simulink model "generic_uservehicle_truck"  (Simulink 8.7)
settings: Solver=ode45  StartTime=0.0  StopTime=inf  RelTol=1e-3
(part 2 of 3)

== system generic_uservehicle_truck/TruckMaker/Vehicle/User Vehicle (ModelMgr)/PowerTrain ==
  note: When replacing the entire powertrain,
      | be sure to disable the IPG powertrain model by using the powertrain
      | model 'Model Manager off' in the vehicle GUI.
  note: <Your model here>
  Sync_In : Inport
  Vhcl.Wheel.PT : Inport  Port=2
  VhclCtrl.PT : Inport  Port=3
  BusCreator : BusCreator  Inputs=70
  Demux : Demux  Outputs=70
  PowerTrain : S-Function  FunctionName=TM_Sfun  Parameters='PowerTrain'  SFunctionDeploymentMode=off  EnableBusSupport=off
  PowerTrainUpd : S-Function  FunctionName=TM_Sfun  Parameters='PowerTrainUpd'  SFunctionDeploymentMode=off  EnableBusSupport=off
  Sync_Out : Outport
  wires:
  Demux/70 -> BusCreator/70  "PT IF WFR2 Trq_BrakeReg_max"
  Demux/69 -> BusCreator/69  "PT IF WFR2 Trq_BrakeReg"
  Demux/68 -> BusCreator/68  "PT IF WFR2 Trq_Supp2WC"
  Demux/67 -> BusCreator/67  "PT IF WFR2 Trq_Drive"
  Demux/66 -> BusCreator/66  "PT IF WFR2 Trq_B2W"
  Demux/65 -> BusCreator/65  "PT IF WFR2 rotv"
  Demux/64 -> BusCreator/64  "PT IF WFR2 rot"
  Demux/63 -> BusCreator/63  "PT IF WFL2 Trq_BrakeReg_max"
  Demux/62 -> BusCreator/62  "PT IF WFL2 Trq_BrakeReg"
  Demux/61 -> BusCreator/61  "PT IF WFL2 Trq_Supp2WC"
  Demux/60 -> BusCreator/60  "PT IF WFL2 Trq_Drive"
  Demux/59 -> BusCreator/59  "PT IF WFL2 Trq_B2W"
  Demux/58 -> BusCreator/58  "PT IF WFL2 rotv"
  Demux/57 -> BusCreator/57  "PT IF WFL2 rot"
  Demux/56 -> BusCreator/56  "PT IF WRR2 Trq_BrakeReg_max"
  Demux/55 -> BusCreator/55  "PT IF WRR2 Trq_BrakeReg"
  Demux/54 -> BusCreator/54  "PT IF WRR2 Trq_Supp2WC"
  Demux/53 -> BusCreator/53  "PT IF WRR2 Trq_Drive"
  Demux/52 -> BusCreator/52  "PT IF WRR2 Trq_B2W"
  Demux/51 -> BusCreator/51  "PT IF WRR2 rotv"
  Demux/50 -> BusCreator/50  "PT IF WRR2 rot"
  Demux/49 -> BusCreator/49  "PT IF WRL2 Trq_BrakeReg_max"
  Demux/48 -> BusCreator/48  "PT IF WRL2 Trq_BrakeReg"
  Demux/47 -> BusCreator/47  "PT IF WRL2 Trq_Supp2WC"
  Demux/46 -> BusCreator/46  "PT IF WRL2 Trq_Drive"
  Demux/45 -> BusCreator/45  "PT IF WRL2 Trq_B2W"
  Demux/44 -> BusCreator/44  "PT IF WRL2 rotv"
  Demux/43 -> BusCreator/43  "PT IF WRL2 rot"
  Demux/42 -> BusCreator/42  "PT IF WRR Trq_BrakeReg_max"
  Demux/41 -> BusCreator/41  "PT IF WRR Trq_BrakeReg"
  Demux/40 -> BusCreator/40  "PT IF WRR Trq_Supp2WC"
  Demux/39 -> BusCreator/39  "PT IF WRR Trq_Drive"
  Demux/38 -> BusCreator/38  "PT IF WRR Trq_B2W"
  Demux/37 -> BusCreator/37  "PT IF WRR rotv"
  Demux/36 -> BusCreator/36  "PT IF WRR rot"
  Demux/35 -> BusCreator/35  "PT IF WRL Trq_BrakeReg_max"
  Demux/34 -> BusCreator/34  "PT IF WRL Trq_BrakeReg"
  Demux/33 -> BusCreator/33  "PT IF WRL Trq_Supp2WC"
  Demux/32 -> BusCreator/32  "PT IF WRL Trq_Drive"
  Demux/31 -> BusCreator/31  "PT IF WRL Trq_B2W"
  Demux/30 -> BusCreator/30  "PT IF WRL rotv"
  Demux/29 -> BusCreator/29  "PT IF WRL rot"
  Demux/28 -> BusCreator/28  "PT IF WFR Trq_BrakeReg_max"
  Demux/27 -> BusCreator/27  "PT IF WFR Trq_BrakeReg"
  Demux/26 -> BusCreator/26  "PT IF WFR Trq_Supp2WC"
  Demux/25 -> BusCreator/25  "PT IF WFR Trq_Drive"
  Demux/24 -> BusCreator/24  "PT IF WFR Trq_B2W"
  Demux/23 -> BusCreator/23  "PT IF WFR rotv"
  Demux/22 -> BusCreator/22  "PT IF WFR rot"
  Demux/21 -> BusCreator/21  "PT IF WFL Trq_BrakeReg_max"
  Demux/20 -> BusCreator/20  "PT IF WFL Trq_BrakeReg"
  Demux/19 -> BusCreator/19  "PT IF WFL Trq_Supp2WC"
  Demux/18 -> BusCreator/18  "PT IF WFL Trq_Drive"
  Demux/17 -> BusCreator/17  "PT IF WFL Trq_B2W"
  Demux/16 -> BusCreator/16  "PT IF WFL rotv"
  Demux/15 -> BusCreator/15  "PT IF WFL rot"
  Demux/14 -> BusCreator/14  "PT IF DL_iDiff_mean"
  Demux/13 -> BusCreator/13  "PT IF Trq_Supp2BdyEng y"
  Demux/12 -> BusCreator/12  "PT IF Trq_Supp2BdyEng x"
  Demux/11 -> BusCreator/11  "PT IF Trq_Supp2Bdy1B z"
  Demux/10 -> BusCreator/10  "PT IF Trq_Supp2Bdy1B y"
  Demux/9 -> BusCreator/9  "PT IF Trq_Supp2Bdy1B x"
  Demux/8 -> BusCreator/8  "PT IF Trq_Supp2Bdy1 z"
  Demux/7 -> BusCreator/7  "PT IF Trq_Supp2Bdy1 y"
  Demux/6 -> BusCreator/6  "PT IF Trq_Supp2Bdy1 x"
  Demux/5 -> BusCreator/5  "PT IF Engine_rotv"
  Demux/4 -> BusCreator/4  "PT IF GearNo"
  Demux/3 -> BusCreator/3  "PT IF OperationError"
  Demux/2 -> BusCreator/2  "PT IF OperationState"
  Demux/1 -> BusCreator/1  "PT IF Ignition"
  BusCreator/1 -> PowerTrainUpd/2
  PowerTrain/2 -> Demux/1
  Sync_In/1 -> PowerTrain/1
  PowerTrainUpd/1 -> Sync_Out/1
  PowerTrain/1 -> PowerTrainUpd/1  "Sync"
  VhclCtrl.PT/1 -> PowerTrain/3
  Vhcl.Wheel.PT/1 -> PowerTrain/2

== system generic_uservehicle_truck/TruckMaker/Vehicle/User Vehicle (ModelMgr)/VehicleSource_ModelMgr ==
  u : Inport
  Compare : RelationalOperator  Operator=~=  OutDataTypeStr=boolean  ZeroCross=off  InputSameDT=on
  Constant : Constant  DisableCoverage=on  Value=const  OutDataTypeStr=Inherit: Inherit via back propagation
  y : Outport
  wires:
  u/1 -> Compare/1
  Constant/1 -> Compare/2
  Compare/1 -> y/1

== system generic_uservehicle_truck/TruckMaker/Vehicle/IPG Vehicle/Brake/CreateBus Vhcl.Wheel.PT ==
  In : Inport
  BusCreator : BusCreator  Inputs=40
  Demux : Demux  Outputs=40
  Out : Outport
  wires:
  Demux/40 -> BusCreator/40  "Vhcl Trq_DriveSrc_trg d7"
  Demux/39 -> BusCreator/39  "Vhcl Trq_DriveSrc_trg d6"
  Demux/38 -> BusCreator/38  "Vhcl Trq_DriveSrc_trg d5"
  Demux/37 -> BusCreator/37  "Vhcl Trq_DriveSrc_trg d4"
  Demux/36 -> BusCreator/36  "Vhcl Trq_DriveSrc_trg d3"
  Demux/35 -> BusCreator/35  "Vhcl Trq_DriveSrc_trg d2"
  Demux/34 -> BusCreator/34  "Vhcl Trq_DriveSrc_trg d1"
  Demux/33 -> BusCreator/33  "Vhcl Trq_DriveSrc_trg d0"
  Demux/32 -> BusCreator/32  "Vhcl Wheel FR2 WhlBearing"
  Demux/31 -> BusCreator/31  "Vhcl Wheel FR2 Trq_T2W"
  Demux/30 -> BusCreator/30  "Vhcl Wheel FR2 Trq_BrakeReg_trg"
  Demux/29 -> BusCreator/29  "Vhcl Wheel FR2 Trq_Brake"
  Demux/28 -> BusCreator/28  "Vhcl Wheel FL2 WhlBearing"
  Demux/27 -> BusCreator/27  "Vhcl Wheel FL2 Trq_T2W"
  Demux/26 -> BusCreator/26  "Vhcl Wheel FL2 Trq_BrakeReg_trg"
  Demux/25 -> BusCreator/25  "Vhcl Wheel FL2 Trq_Brake"
  Demux/24 -> BusCreator/24  "Vhcl Wheel RR2 WhlBearing"
  Demux/23 -> BusCreator/23  "Vhcl Wheel RR2 Trq_T2W"
  Demux/22 -> BusCreator/22  "Vhcl Wheel RR2 Trq_BrakeReg_trg"
  Demux/21 -> BusCreator/21  "Vhcl Wheel RR2 Trq_Brake"
  Demux/20 -> BusCreator/20  "Vhcl Wheel RL2 WhlBearing"
  Demux/19 -> BusCreator/19  "Vhcl Wheel RL2 Trq_T2W"
  Demux/18 -> BusCreator/18  "Vhcl Wheel RL2 Trq_BrakeReg_trg"
  Demux/17 -> BusCreator/17  "Vhcl Wheel RL2 Trq_Brake"
  Demux/16 -> BusCreator/16  "Vhcl Wheel RR WhlBearing"
  Demux/15 -> BusCreator/15  "Vhcl Wheel RR Trq_T2W"
  Demux/14 -> BusCreator/14  "Vhcl Wheel RR Trq_BrakeReg_trg"
  Demux/13 -> BusCreator/13  "Vhcl Wheel RR Trq_Brake"
  Demux/12 -> BusCreator/12  "Vhcl Wheel RL WhlBearing"
  Demux/11 -> BusCreator/11  "Vhcl Wheel RL Trq_T2W"
  Demux/10 -> BusCreator/10  "Vhcl Wheel RL Trq_BrakeReg_trg"
  Demux/9 -> BusCreator/9  "Vhcl Wheel RL Trq_Brake"
  Demux/8 -> BusCreator/8  "Vhcl Wheel FR WhlBearing"
  Demux/7 -> BusCreator/7  "Vhcl Wheel FR Trq_T2W"
  Demux/6 -> BusCreator/6  "Vhcl Wheel FR Trq_BrakeReg_trg"
  Demux/5 -> BusCreator/5  "Vhcl Wheel FR Trq_Brake"
  Demux/4 -> BusCreator/4  "Vhcl Wheel FL WhlBearing"
  Demux/3 -> BusCreator/3  "Vhcl Wheel FL Trq_T2W"
  Demux/2 -> BusCreator/2  "Vhcl Wheel FL Trq_BrakeReg_trg"
  Demux/1 -> BusCreator/1  "Vhcl Wheel FL Trq_Brake"
  BusCreator/1 -> Out/1
  In/1 -> Demux/1

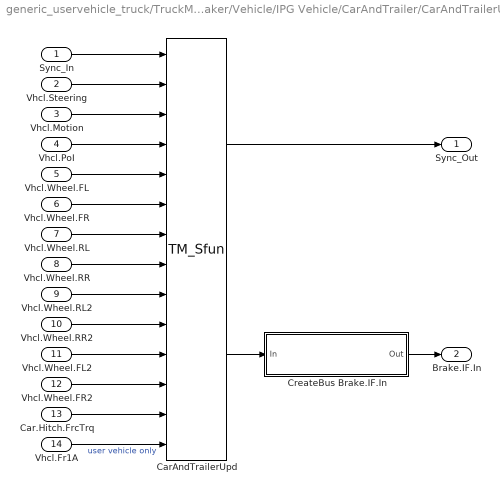
== system generic_uservehicle_truck/TruckMaker/Vehicle/IPG Vehicle/CarAndTrailer/CarAndTrailerUpd ==
  Sync_In : Inport
  Vhcl.Steering : Inport  Port=2
  Vhcl.Motion : Inport  Port=3
  Vhcl.PoI : Inport  Port=4
  Vhcl.Wheel.FL : Inport  Port=5
  Vhcl.Wheel.FR : Inport  Port=6
  Vhcl.Wheel.RL : Inport  Port=7
  Vhcl.Wheel.RR : Inport  Port=8
  Vhcl.Wheel.RL2 : Inport  Port=9
  Vhcl.Wheel.RR2 : Inport  Port=10
  Vhcl.Wheel.FL2 : Inport  Port=11
  Vhcl.Wheel.FR2 : Inport  Port=12
  Car.Hitch.FrcTrq : Inport  Port=13
  Vhcl.Fr1A : Inport  Port=14
  CarAndTrailerUpd : S-Function  FunctionName=TM_Sfun  Parameters='CarAndTrUpd'  SFunctionDeploymentMode=off  EnableBusSupport=off
  CreateBus Brake.IF.In : Subsystem
  Sync_Out : Outport
  Brake.IF.In : Outport  Port=2
  wires:
  Vhcl.Fr1A/1 -> CarAndTrailerUpd/14  "user vehicle only"
  Vhcl.Wheel.RL2/1 -> CarAndTrailerUpd/9
  Vhcl.Wheel.RR2/1 -> CarAndTrailerUpd/10
  Vhcl.Wheel.FL2/1 -> CarAndTrailerUpd/11
  Vhcl.Wheel.FR2/1 -> CarAndTrailerUpd/12
  Car.Hitch.FrcTrq/1 -> CarAndTrailerUpd/13
  Vhcl.Wheel.RR/1 -> CarAndTrailerUpd/8
  Vhcl.Wheel.RL/1 -> CarAndTrailerUpd/7
  Vhcl.Wheel.FR/1 -> CarAndTrailerUpd/6
  Vhcl.Wheel.FL/1 -> CarAndTrailerUpd/5
  Vhcl.Steering/1 -> CarAndTrailerUpd/2
  Vhcl.Motion/1 -> CarAndTrailerUpd/3
  Vhcl.PoI/1 -> CarAndTrailerUpd/4
  CarAndTrailerUpd/2 -> CreateBus Brake.IF.In/1(In)
  CreateBus Brake.IF.In/1(Out) -> Brake.IF.In/1
  CarAndTrailerUpd/1 -> Sync_Out/1
  Sync_In/1 -> CarAndTrailerUpd/1

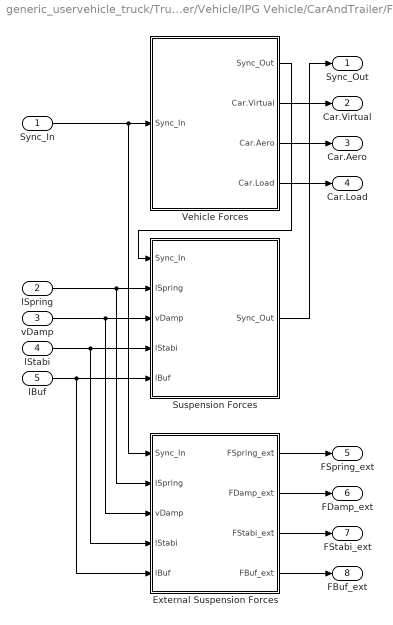
== system generic_uservehicle_truck/TruckMaker/Vehicle/IPG Vehicle/CarAndTrailer/Forces ==
  Sync_In : Inport
  lSpring : Inport  Port=2
  vDamp : Inport  Port=3
  lStabi : Inport  Port=4
  lBuf : Inport  Port=5
  External Suspension Forces : Subsystem
  Suspension Forces : Subsystem
  Vehicle Forces : Subsystem
  Sync_Out : Outport
  Car.Virtual : Outport  Port=2
  Car.Aero : Outport  Port=3
  Car.Load : Outport  Port=4
  FSpring_ext : Outport  Port=5
  FDamp_ext : Outport  Port=6
  FStabi_ext : Outport  Port=7
  FBuf_ext : Outport  Port=8
  wires:
  Sync_In/1 -> External Suspension Forces/1(Sync_In), Vehicle Forces/1(Sync_In)
  Vehicle Forces/2(Car.Virtual) -> Car.Virtual/1
  Vehicle Forces/3(Car.Aero) -> Car.Aero/1
  Vehicle Forces/4(Car.Load) -> Car.Load/1
  lSpring/1 -> Suspension Forces/2(lSpring), External Suspension Forces/2(lSpring)
  External Suspension Forces/2(FDamp_ext) -> FDamp_ext/1
  vDamp/1 -> Suspension Forces/3(vDamp), External Suspension Forces/3(vDamp)
  lStabi/1 -> Suspension Forces/4(lStabi), External Suspension Forces/4(lStabi)
  External Suspension Forces/3(FStabi_ext) -> FStabi_ext/1
  External Suspension Forces/1(FSpring_ext) -> FSpring_ext/1
  lBuf/1 -> Suspension Forces/5(lBuf), External Suspension Forces/5(lBuf)
  External Suspension Forces/4(FBuf_ext) -> FBuf_ext/1
  Vehicle Forces/1(Sync_Out) -> Suspension Forces/1(Sync_In)
  Suspension Forces/1(Sync_Out) -> Sync_Out/1

== system generic_uservehicle_truck/TruckMaker/Vehicle/IPG Vehicle/CarAndTrailer/Kinematics ==
  Sync_In : Inport
  Steer.IF : Inport  Port=2
  Kinematics : S-Function  FunctionName=TM_Sfun  Parameters='Kinematics'  SFunctionDeploymentMode=off  EnableBusSupport=off
  TireFL.In : Terminator
  TireFR.In : Terminator
  TireRL.In : Terminator
  TireRR.In : Terminator
  Sync_Out : Outport
  lSpring : Outport  Port=2
  vDamp : Outport  Port=3
  lStabi : Outport  Port=4
  lBuf : Outport  Port=5
  wires:
  Kinematics/8 -> lStabi/1
  Kinematics/2 -> TireFL.In/1
  Kinematics/3 -> TireFR.In/1
  Kinematics/4 -> TireRL.In/1
  Kinematics/5 -> TireRR.In/1
  Kinematics/6 -> lSpring/1
  Kinematics/7 -> vDamp/1
  Sync_In/1 -> Kinematics/1
  Kinematics/1 -> Sync_Out/1
  Steer.IF/1 -> Kinematics/2
  Kinematics/9 -> lBuf/1

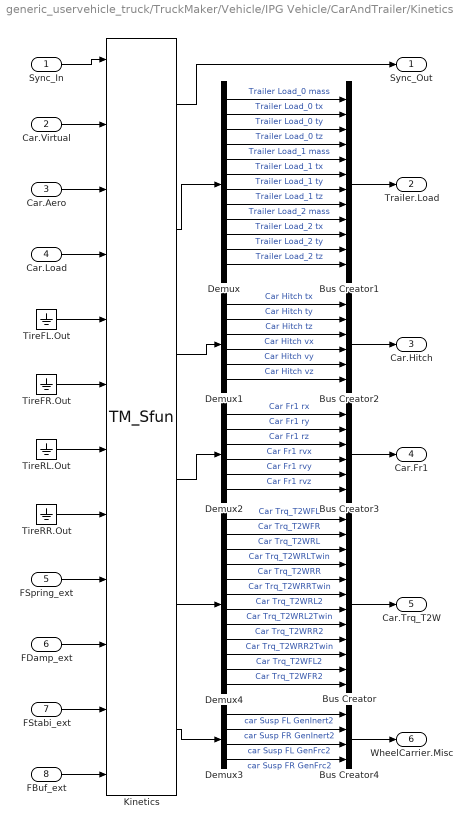
== system generic_uservehicle_truck/TruckMaker/Vehicle/IPG Vehicle/CarAndTrailer/Kinetics ==
  Sync_In : Inport
  Car.Virtual : Inport  Port=2
  Car.Aero : Inport  Port=3
  Car.Load : Inport  Port=4
  FSpring_ext : Inport  Port=5
  FDamp_ext : Inport  Port=6
  FStabi_ext : Inport  Port=7
  FBuf_ext : Inport  Port=8
  Bus Creator : BusCreator  Inputs=12
  Bus Creator1 : BusCreator  Inputs=12
  Bus Creator2 : BusCreator  Inputs=6
  Bus Creator3 : BusCreator  Inputs=6
  Bus Creator4 : BusCreator  Inputs=4
  Demux : Demux  Outputs=12
  Demux1 : Demux  Outputs=6
  Demux2 : Demux  Outputs=6
  Demux3 : Demux
  Demux4 : Demux  Outputs=12
  Kinetics : S-Function  FunctionName=TM_Sfun  Parameters='Kinetics'  SFunctionDeploymentMode=off  EnableBusSupport=off
  TireFL.Out : Ground
  TireFR.Out : Ground
  TireRL.Out : Ground
  TireRR.Out : Ground
  Sync_Out : Outport
  Trailer.Load : Outport  Port=2
  Car.Hitch : Outport  Port=3
  Car.Fr1 : Outport  Port=4
  Car.Trq_T2W : Outport  Port=5
  WheelCarrier.Misc : Outport  Port=6
  wires:
  Demux4/12 -> Bus Creator/12  "Car Trq_T2WFR2"
  Demux4/11 -> Bus Creator/11  "Car Trq_T2WFL2"
  Sync_In/1 -> Kinetics/1
  Kinetics/1 -> Sync_Out/1
  Car.Aero/1 -> Kinetics/3
  Car.Virtual/1 -> Kinetics/2
  Bus Creator1/1 -> Trailer.Load/1
  Demux/1 -> Bus Creator1/1  "Trailer Load_0 mass"
  Demux/2 -> Bus Creator1/2  "Trailer Load_0 tx"
  Demux/3 -> Bus Creator1/3  "Trailer Load_0 ty"
  Demux/4 -> Bus Creator1/4  "Trailer Load_0 tz"
  Kinetics/2 -> Demux/1
  Demux/5 -> Bus Creator1/5  "Trailer Load_1 mass"
  Demux/6 -> Bus Creator1/6  "Trailer Load_1 tx"
  Demux/7 -> Bus Creator1/7  "Trailer Load_1 ty"
  Demux/8 -> Bus Creator1/8  "Trailer Load_1 tz"
  Demux/9 -> Bus Creator1/9  "Trailer Load_2 mass"
  Demux/10 -> Bus Creator1/10  "Trailer Load_2 tx"
  Demux/11 -> Bus Creator1/11  "Trailer Load_2 ty"
  Demux/12 -> Bus Creator1/12  "Trailer Load_2 tz"
  Demux1/1 -> Bus Creator2/1  "Car Hitch tx"
  Demux1/2 -> Bus Creator2/2  "Car Hitch ty"
  Demux1/3 -> Bus Creator2/3  "Car Hitch tz"
  Demux1/4 -> Bus Creator2/4  "Car Hitch vx"
  Demux1/5 -> Bus Creator2/5  "Car Hitch vy"
  Demux1/6 -> Bus Creator2/6  "Car Hitch vz"
  Kinetics/3 -> Demux1/1
  Bus Creator2/1 -> Car.Hitch/1
  Demux2/1 -> Bus Creator3/1  "Car Fr1 rx"
  Demux2/2 -> Bus Creator3/2  "Car Fr1 ry"
  Demux2/3 -> Bus Creator3/3  "Car Fr1 rz"
  Demux2/4 -> Bus Creator3/4  "Car Fr1 rvx"
  Demux2/5 -> Bus Creator3/5  "Car Fr1 rvy"
  Demux2/6 -> Bus Creator3/6  "Car Fr1 rvz"
  Bus Creator3/1 -> Car.Fr1/1
  Kinetics/4 -> Demux2/1
  Car.Load/1 -> Kinetics/4
  Demux3/1 -> Bus Creator4/1  "car Susp FL GenInert2"
  Demux3/2 -> Bus Creator4/2  "car Susp FR GenInert2"
  Demux3/3 -> Bus Creator4/3  "car Susp FL GenFrc2"
  Demux3/4 -> Bus Creator4/4  "car Susp FR GenFrc2"
  Bus Creator4/1 -> WheelCarrier.Misc/1
  Demux4/3 -> Bus Creator/3  "Car Trq_T2WRL"
  Demux4/2 -> Bus Creator/2  "Car Trq_T2WFR"
  Demux4/1 -> Bus Creator/1  "Car Trq_T2WFL"
  TireFL.Out/1 -> Kinetics/5
  TireFR.Out/1 -> Kinetics/6
  TireRL.Out/1 -> Kinetics/7
  TireRR.Out/1 -> Kinetics/8
  FSpring_ext/1 -> Kinetics/9
  FDamp_ext/1 -> Kinetics/10
  FStabi_ext/1 -> Kinetics/11
  Kinetics/6 -> Demux3/1
  Kinetics/5 -> Demux4/1
  Bus Creator/1 -> Car.Trq_T2W/1
  Demux4/9 -> Bus Creator/9  "Car Trq_T2WRR2"
  Demux4/10 -> Bus Creator/10  "Car Trq_T2WRR2Twin"
  Demux4/7 -> Bus Creator/7  "Car Trq_T2WRL2"
  Demux4/8 -> Bus Creator/8  "Car Trq_T2WRL2Twin"
  Demux4/5 -> Bus Creator/5  "Car Trq_T2WRR"
  Demux4/4 -> Bus Creator/4  "Car Trq_T2WRLTwin"
  Demux4/6 -> Bus Creator/6  "Car Trq_T2WRRTwin"
  FBuf_ext/1 -> Kinetics/12

== system generic_uservehicle_truck/TruckMaker/Vehicle/IPG Vehicle/CarAndTrailer/Steering ==
  note: When replacing the entire steering system,
      | be sure to disable the IPG steering model by using the steering
      | model 'Model Manager off' in the vehicle GUI.
  Sync_In : Inport
  VhclCtrl.Steering : Inport  Port=2
  Bus Creator1 : BusCreator  Inputs=16
  Bus Creator2 : BusCreator  Inputs=5
  Demux : Demux  Outputs=21
  Steering : S-Function  FunctionName=TM_Sfun  Parameters='Steering'  SFunctionDeploymentMode=off  EnableBusSupport=off
  Terminator : Terminator
  Sync_Out : Outport
  Steer.IF : Outport  Port=2
  wires:
  Demux/21 -> Bus Creator2/5  "Steering IF R Inert"
  Demux/20 -> Bus Creator2/4  "Steering IF R Frc"
  Demux/19 -> Bus Creator2/3  "Steering IF L Inert"
  Demux/18 -> Bus Creator2/2  "Steering IF L Frc"
  Demux/17 -> Bus Creator2/1  "Steering IF SteerByTrq"
  Demux/16 -> Bus Creator1/16  "Steering IF R iSteer2q"
  Demux/15 -> Bus Creator1/15  "Steering IF R qpp"
  Demux/14 -> Bus Creator1/14  "Steering IF R qp"
  Demux/13 -> Bus Creator1/13  "Steering IF R q"
  Demux/12 -> Bus Creator1/12  "Steering IF L iSteer2q"
  Demux/11 -> Bus Creator1/11  "Steering IF L qpp"
  Demux/10 -> Bus Creator1/10  "Steering IF L qp"
  Demux/9 -> Bus Creator1/9  "Steering IF L q"
  Demux/8 -> Bus Creator1/8  "Steering IF AssistTrqPin"
  Demux/7 -> Bus Creator1/7  "Steering IF AssistTrqCol"
  Demux/6 -> Bus Creator1/6  "Steering IF AssistFrc"
  Demux/5 -> Bus Creator1/5  "Steering IF TrqStatic"
  Demux/4 -> Bus Creator1/4  "Steering IF Trq"
  Demux/3 -> Bus Creator1/3  "Steering IF AngAcc"
  Demux/2 -> Bus Creator1/2  "Steering IF AngVel"
  Demux/1 -> Bus Creator1/1  "Steering IF Ang"
  Bus Creator1/1 -> Steer.IF/1
  Bus Creator2/1 -> Terminator/1  "Steer IF (in)"
  Sync_In/1 -> Steering/1
  Steering/1 -> Sync_Out/1
  VhclCtrl.Steering/1 -> Steering/2
  Steering/2 -> Demux/1

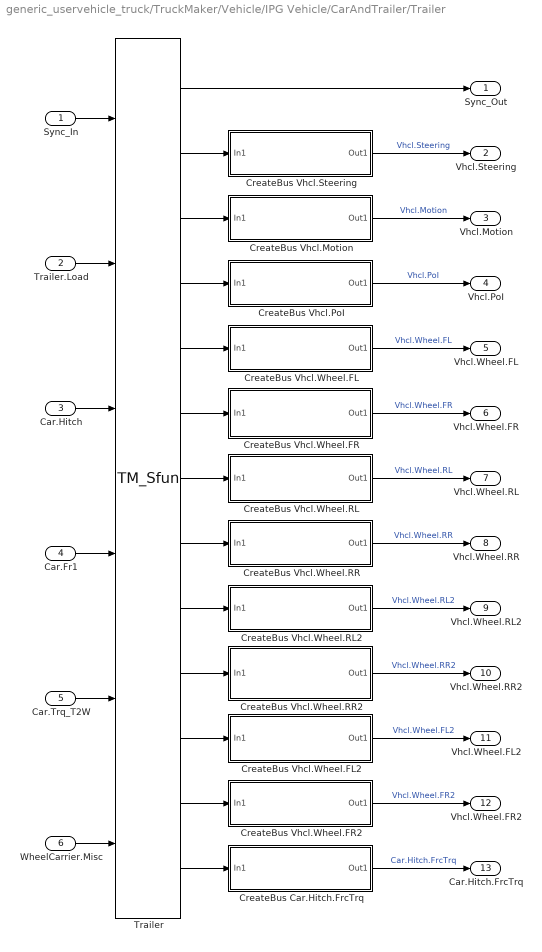
== system generic_uservehicle_truck/TruckMaker/Vehicle/IPG Vehicle/CarAndTrailer/Trailer ==
  Sync_In : Inport
  Trailer.Load : Inport  Port=2
  Car.Hitch : Inport  Port=3
  Car.Fr1 : Inport  Port=4
  Car.Trq_T2W : Inport  Port=5
  WheelCarrier.Misc : Inport  Port=6
  CreateBus Car.Hitch.FrcTrq : Subsystem
  CreateBus Vhcl.Motion : Subsystem
  CreateBus Vhcl.PoI : Subsystem
  CreateBus Vhcl.Steering : Subsystem
  CreateBus Vhcl.Wheel.FL : Subsystem
  CreateBus Vhcl.Wheel.FL2 : Subsystem
  CreateBus Vhcl.Wheel.FR : Subsystem
  CreateBus Vhcl.Wheel.FR2 : Subsystem
  CreateBus Vhcl.Wheel.RL : Subsystem
  CreateBus Vhcl.Wheel.RL2 : Subsystem
  CreateBus Vhcl.Wheel.RR : Subsystem
  CreateBus Vhcl.Wheel.RR2 : Subsystem
  Trailer : S-Function  FunctionName=TM_Sfun  Parameters='Trailer'  SFunctionDeploymentMode=off  EnableBusSupport=off
  Sync_Out : Outport
  Vhcl.Steering : Outport  Port=2
  Vhcl.Motion : Outport  Port=3
  Vhcl.PoI : Outport  Port=4
  Vhcl.Wheel.FL : Outport  Port=5
  Vhcl.Wheel.FR : Outport  Port=6
  Vhcl.Wheel.RL : Outport  Port=7
  Vhcl.Wheel.RR : Outport  Port=8
  Vhcl.Wheel.RL2 : Outport  Port=9
  Vhcl.Wheel.RR2 : Outport  Port=10
  Vhcl.Wheel.FL2 : Outport  Port=11
  Vhcl.Wheel.FR2 : Outport  Port=12
  Car.Hitch.FrcTrq : Outport  Port=13
  wires:
  CreateBus Vhcl.Wheel.RL2/1(Out1) -> Vhcl.Wheel.RL2/1  "Vhcl.Wheel.RL2"
  CreateBus Vhcl.Wheel.RR2/1(Out1) -> Vhcl.Wheel.RR2/1  "Vhcl.Wheel.RR2"
  CreateBus Vhcl.Wheel.FL2/1(Out1) -> Vhcl.Wheel.FL2/1  "Vhcl.Wheel.FL2"
  CreateBus Vhcl.Wheel.FR2/1(Out1) -> Vhcl.Wheel.FR2/1  "Vhcl.Wheel.FR2"
  Trailer/12 -> CreateBus Vhcl.Wheel.FR2/1(In1)
  Trailer/11 -> CreateBus Vhcl.Wheel.FL2/1(In1)
  Trailer/10 -> CreateBus Vhcl.Wheel.RR2/1(In1)
  Trailer/9 -> CreateBus Vhcl.Wheel.RL2/1(In1)
  CreateBus Vhcl.Wheel.FL/1(Out1) -> Vhcl.Wheel.FL/1  "Vhcl.Wheel.FL"
  CreateBus Vhcl.Wheel.FR/1(Out1) -> Vhcl.Wheel.FR/1  "Vhcl.Wheel.FR"
  CreateBus Vhcl.Wheel.RL/1(Out1) -> Vhcl.Wheel.RL/1  "Vhcl.Wheel.RL"
  CreateBus Vhcl.Wheel.RR/1(Out1) -> Vhcl.Wheel.RR/1  "Vhcl.Wheel.RR"
  Trailer/8 -> CreateBus Vhcl.Wheel.RR/1(In1)
  Trailer/7 -> CreateBus Vhcl.Wheel.RL/1(In1)
  Trailer/6 -> CreateBus Vhcl.Wheel.FR/1(In1)
  Trailer/5 -> CreateBus Vhcl.Wheel.FL/1(In1)
  Trailer/13 -> CreateBus Car.Hitch.FrcTrq/1(In1)
  Trailer/2 -> CreateBus Vhcl.Steering/1(In1)
  CreateBus Vhcl.Steering/1(Out1) -> Vhcl.Steering/1  "Vhcl.Steering"
  Trailer/3 -> CreateBus Vhcl.Motion/1(In1)
  Trailer/4 -> CreateBus Vhcl.PoI/1(In1)
  CreateBus Vhcl.PoI/1(Out1) -> Vhcl.PoI/1  "Vhcl.PoI"
  CreateBus Vhcl.Motion/1(Out1) -> Vhcl.Motion/1  "Vhcl.Motion"
  Car.Trq_T2W/1 -> Trailer/5
  WheelCarrier.Misc/1 -> Trailer/6
  CreateBus Car.Hitch.FrcTrq/1(Out1) -> Car.Hitch.FrcTrq/1  "Car.Hitch.FrcTrq"
  Car.Fr1/1 -> Trailer/4
  Car.Hitch/1 -> Trailer/3
  Trailer.Load/1 -> Trailer/2
  Trailer/1 -> Sync_Out/1
  Sync_In/1 -> Trailer/1

== system generic_uservehicle_truck/TruckMaker/Vehicle/User Vehicle (CM4SL)/Brake/CreateBus Vhcl.Wheel.PT ==
  In : Inport
  BusCreator : BusCreator  Inputs=40
  Demux : Demux  Outputs=40
  Out : Outport
  wires:
  Demux/40 -> BusCreator/40  "Vhcl Trq_DriveSrc_trg d7"
  Demux/39 -> BusCreator/39  "Vhcl Trq_DriveSrc_trg d6"
  Demux/38 -> BusCreator/38  "Vhcl Trq_DriveSrc_trg d5"
  Demux/37 -> BusCreator/37  "Vhcl Trq_DriveSrc_trg d4"
  Demux/36 -> BusCreator/36  "Vhcl Trq_DriveSrc_trg d3"
  Demux/35 -> BusCreator/35  "Vhcl Trq_DriveSrc_trg d2"
  Demux/34 -> BusCreator/34  "Vhcl Trq_DriveSrc_trg d1"
  Demux/33 -> BusCreator/33  "Vhcl Trq_DriveSrc_trg d0"
  Demux/32 -> BusCreator/32  "Vhcl Wheel FR2 WhlBearing"
  Demux/31 -> BusCreator/31  "Vhcl Wheel FR2 Trq_T2W"
  Demux/30 -> BusCreator/30  "Vhcl Wheel FR2 Trq_BrakeReg_trg"
  Demux/29 -> BusCreator/29  "Vhcl Wheel FR2 Trq_Brake"
  Demux/28 -> BusCreator/28  "Vhcl Wheel FL2 WhlBearing"
  Demux/27 -> BusCreator/27  "Vhcl Wheel FL2 Trq_T2W"
  Demux/26 -> BusCreator/26  "Vhcl Wheel FL2 Trq_BrakeReg_trg"
  Demux/25 -> BusCreator/25  "Vhcl Wheel FL2 Trq_Brake"
  Demux/24 -> BusCreator/24  "Vhcl Wheel RR2 WhlBearing"
  Demux/23 -> BusCreator/23  "Vhcl Wheel RR2 Trq_T2W"
  Demux/22 -> BusCreator/22  "Vhcl Wheel RR2 Trq_BrakeReg_trg"
  Demux/21 -> BusCreator/21  "Vhcl Wheel RR2 Trq_Brake"
  Demux/20 -> BusCreator/20  "Vhcl Wheel RL2 WhlBearing"
  Demux/19 -> BusCreator/19  "Vhcl Wheel RL2 Trq_T2W"
  Demux/18 -> BusCreator/18  "Vhcl Wheel RL2 Trq_BrakeReg_trg"
  Demux/17 -> BusCreator/17  "Vhcl Wheel RL2 Trq_Brake"
  Demux/16 -> BusCreator/16  "Vhcl Wheel RR WhlBearing"
  Demux/15 -> BusCreator/15  "Vhcl Wheel RR Trq_T2W"
  Demux/14 -> BusCreator/14  "Vhcl Wheel RR Trq_BrakeReg_trg"
  Demux/13 -> BusCreator/13  "Vhcl Wheel RR Trq_Brake"
  Demux/12 -> BusCreator/12  "Vhcl Wheel RL WhlBearing"
  Demux/11 -> BusCreator/11  "Vhcl Wheel RL Trq_T2W"
  Demux/10 -> BusCreator/10  "Vhcl Wheel RL Trq_BrakeReg_trg"
  Demux/9 -> BusCreator/9  "Vhcl Wheel RL Trq_Brake"
  Demux/8 -> BusCreator/8  "Vhcl Wheel FR WhlBearing"
  Demux/7 -> BusCreator/7  "Vhcl Wheel FR Trq_T2W"
  Demux/6 -> BusCreator/6  "Vhcl Wheel FR Trq_BrakeReg_trg"
  Demux/5 -> BusCreator/5  "Vhcl Wheel FR Trq_Brake"
  Demux/4 -> BusCreator/4  "Vhcl Wheel FL WhlBearing"
  Demux/3 -> BusCreator/3  "Vhcl Wheel FL Trq_T2W"
  Demux/2 -> BusCreator/2  "Vhcl Wheel FL Trq_BrakeReg_trg"
  Demux/1 -> BusCreator/1  "Vhcl Wheel FL Trq_Brake"
  BusCreator/1 -> Out/1
  In/1 -> Demux/1

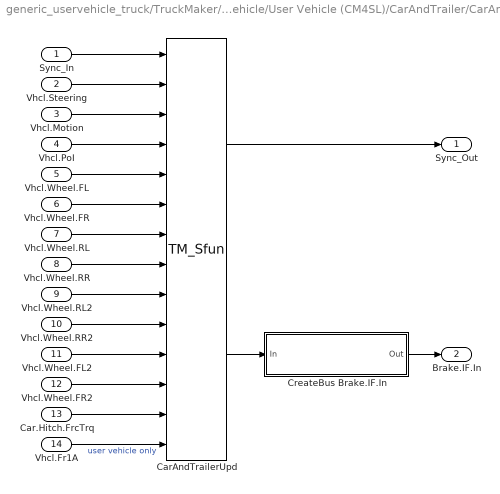
== system generic_uservehicle_truck/TruckMaker/Vehicle/User Vehicle (CM4SL)/CarAndTrailer/CarAndTrailerUpd ==
  Sync_In : Inport
  Vhcl.Steering : Inport  Port=2
  Vhcl.Motion : Inport  Port=3
  Vhcl.PoI : Inport  Port=4
  Vhcl.Wheel.FL : Inport  Port=5
  Vhcl.Wheel.FR : Inport  Port=6
  Vhcl.Wheel.RL : Inport  Port=7
  Vhcl.Wheel.RR : Inport  Port=8
  Vhcl.Wheel.RL2 : Inport  Port=9
  Vhcl.Wheel.RR2 : Inport  Port=10
  Vhcl.Wheel.FL2 : Inport  Port=11
  Vhcl.Wheel.FR2 : Inport  Port=12
  Car.Hitch.FrcTrq : Inport  Port=13
  Vhcl.Fr1A : Inport  Port=14
  CarAndTrailerUpd : S-Function  FunctionName=TM_Sfun  Parameters='CarAndTrUpd'  SFunctionDeploymentMode=off  EnableBusSupport=off
  CreateBus Brake.IF.In : Subsystem
  Sync_Out : Outport
  Brake.IF.In : Outport  Port=2
  wires:
  Vhcl.Fr1A/1 -> CarAndTrailerUpd/14  "user vehicle only"
  Vhcl.Wheel.RL2/1 -> CarAndTrailerUpd/9
  Vhcl.Wheel.RR2/1 -> CarAndTrailerUpd/10
  Vhcl.Wheel.FL2/1 -> CarAndTrailerUpd/11
  Vhcl.Wheel.FR2/1 -> CarAndTrailerUpd/12
  Car.Hitch.FrcTrq/1 -> CarAndTrailerUpd/13
  Vhcl.Wheel.RR/1 -> CarAndTrailerUpd/8
  Vhcl.Wheel.RL/1 -> CarAndTrailerUpd/7
  Vhcl.Wheel.FR/1 -> CarAndTrailerUpd/6
  Vhcl.Wheel.FL/1 -> CarAndTrailerUpd/5
  Vhcl.Steering/1 -> CarAndTrailerUpd/2
  Vhcl.Motion/1 -> CarAndTrailerUpd/3
  Vhcl.PoI/1 -> CarAndTrailerUpd/4
  CarAndTrailerUpd/2 -> CreateBus Brake.IF.In/1(In)
  CreateBus Brake.IF.In/1(Out) -> Brake.IF.In/1
  CarAndTrailerUpd/1 -> Sync_Out/1
  Sync_In/1 -> CarAndTrailerUpd/1

== system generic_uservehicle_truck/TruckMaker/Vehicle/User Vehicle (CM4SL)/CarAndTrailer/CreateBus Car.Hitch.FrcTrq ==
  Demux7 : Demux  Outputs=6
  Ground7 : Ground
  Mux : Mux  Inputs=6
  Car.Hitch.FrcTrq : Outport
  wires:
  Demux7/1 -> Mux/1  "Car Hitch Frc2Car x"
  Demux7/2 -> Mux/2  "Car Hitch Frc2Car y"
  Demux7/3 -> Mux/3  "Car Hitch Frc2Car z"
  Demux7/4 -> Mux/4  "Car Hitch Trq2Car x"
  Demux7/5 -> Mux/5  "Car Hitch Trq2Car y"
  Demux7/6 -> Mux/6  "Car Hitch Trq2Car z"
  Mux/1 -> Car.Hitch.FrcTrq/1
  Ground7/1 -> Demux7/1

== system generic_uservehicle_truck/TruckMaker/Vehicle/User Vehicle (CM4SL)/CarAndTrailer/CreateBus Vhcl.Fr1A ==
  Demux : Demux  Outputs=24
  Ground7 : Ground
  Mux : Mux  Inputs=24
  Vhcl.Fr1A : Outport
  wires:
  Demux/24 -> Mux/24  "Vhcl Fr1A_Tr2Fr0 22"
  Demux/23 -> Mux/23  "Vhcl Fr1A_Tr2Fr0 21"
  Demux/22 -> Mux/22  "Vhcl Fr1A_Tr2Fr0 20"
  Demux/21 -> Mux/21  "Vhcl Fr1A_Tr2Fr0 12"
  Demux/20 -> Mux/20  "Vhcl Fr1A_Tr2Fr0 11"
  Demux/19 -> Mux/19  "Vhcl Fr1A_Tr2Fr0 10"
  Demux/18 -> Mux/18  "Vhcl Fr1A_Tr2Fr0 02"
  Demux/17 -> Mux/17  "Vhcl Fr1A_Tr2Fr0 01"
  Demux/16 -> Mux/16  "Vhcl Fr1A_Tr2Fr0 00"
  Demux/15 -> Mux/15  "Vhcl Fr1A_alpha_0 z"
  Demux/14 -> Mux/14  "Vhcl Fr1A_alpha_0 y"
  Demux/13 -> Mux/13  "Vhcl Fr1A_alpha_0 x"
  Demux/12 -> Mux/12  "Vhcl Fr1A_omega_0 z"
  Demux/11 -> Mux/11  "Vhcl Fr1A_omega_0 y"
  Demux/10 -> Mux/10  "Vhcl Fr1A_omega_0 x"
  Demux/9 -> Mux/9  "Vhcl Fr1A_a_0 z"
  Demux/8 -> Mux/8  "Vhcl Fr1A_a_0 y"
  Demux/7 -> Mux/7  "Vhcl Fr1A_a_0 x"
  Demux/6 -> Mux/6  "Vhcl Fr1A_v_0 z"
  Demux/5 -> Mux/5  "Vhcl Fr1A_v_0 y"
  Demux/4 -> Mux/4  "Vhcl Fr1A_v_0 x"
  Demux/3 -> Mux/3  "Vhcl Fr1A_t_0 z"
  Demux/2 -> Mux/2  "Vhcl Fr1A_t_0 y"
  Demux/1 -> Mux/1  "Vhcl Fr1A _t_0 x"
  Ground7/1 -> Demux/1
  Mux/1 -> Vhcl.Fr1A/1

== system generic_uservehicle_truck/TruckMaker/Vehicle/User Vehicle (CM4SL)/CarAndTrailer/CreateBus Vhcl.Motion ==
  BusCreator : BusCreator  Inputs=15
  Demux : Demux  Outputs=15
  Ground1 : Ground
  Vhcl .Motion : Outport
  wires:
  BusCreator/1 -> Vhcl .Motion/1
  Ground1/1 -> Demux/1
  Demux/1 -> BusCreator/1  "Vhcl v"
  Demux/2 -> BusCreator/2  "Vhcl Distance"
  Demux/3 -> BusCreator/3  "Vhcl sRoad"
  Demux/4 -> BusCreator/4  "Vhcl Hitch_Pos x"
  Demux/5 -> BusCreator/5  "Vhcl Hitch_Pos y"
  Demux/6 -> BusCreator/6  "Vhcl Hitch_Pos z"
  Demux/7 -> BusCreator/7  "Vhcl Roll"
  Demux/8 -> BusCreator/8  "Vhcl RollVel"
  Demux/9 -> BusCreator/9  "Vhcl RollAcc"
  Demux/10 -> BusCreator/10  "Vhcl Pitch"
  Demux/11 -> BusCreator/11  "Vhcl PitchVel"
  Demux/12 -> BusCreator/12  "Vhcl PitchAcc"
  Demux/13 -> BusCreator/13  "Vhcl Yaw"
  Demux/14 -> BusCreator/14  "Vhcl YawVel"
  Demux/15 -> BusCreator/15  "Vhcl YawAcc"

== system generic_uservehicle_truck/TruckMaker/Vehicle/User Vehicle (CM4SL)/CarAndTrailer/CreateBus Vhcl.PoI ==
  Demux3 : Demux  Outputs=18
  Ground2 : Ground
  Mux : Mux  Inputs=18
  Vhcl.PoI : Outport
  wires:
  Demux3/1 -> Mux/1  "Vhcl PoI_Pos x"
  Mux/1 -> Vhcl.PoI/1
  Ground2/1 -> Demux3/1
  Demux3/2 -> Mux/2  "Vhcl PoI_Pos y"
  Demux3/3 -> Mux/3  "Vhcl PoI_Pos z"
  Demux3/4 -> Mux/4  "Vhcl PoI_Vel x"
  Demux3/5 -> Mux/5  "Vhcl PoI_Vel y"
  Demux3/6 -> Mux/6  "Vhcl PoI_Vel z"
  Demux3/7 -> Mux/7  "Vhcl PoI_Acc x"
  Demux3/8 -> Mux/8  "Vhcl PoI_Acc y"
  Demux3/9 -> Mux/9  "Vhcl PoI_Acc z"
  Demux3/10 -> Mux/10  "Vhcl PoI_Vel_1 x"
  Demux3/11 -> Mux/11  "Vhcl PoI_Vel_1 y"
  Demux3/12 -> Mux/12  "Vhcl PoI_Vel_1 z"
  Demux3/13 -> Mux/13  "Vhcl PoI_Acc_1 x"
  Demux3/14 -> Mux/14  "Vhcl PoI_Acc_1 y"
  Demux3/15 -> Mux/15  "Vhcl PoI_Acc_1 z"
  Demux3/16 -> Mux/16  "Vhcl PoI_GCS Long"
  Demux3/17 -> Mux/17  "Vhcl PoI_GCS Lat"
  Demux3/18 -> Mux/18  "Vhcl PoI_GCS Elev"

== system generic_uservehicle_truck/TruckMaker/Vehicle/User Vehicle (CM4SL)/CarAndTrailer/CreateBus Vhcl.Steering ==
  Demux : Demux
  Ground7 : Ground
  Mux : Mux
  Vhcl.Steering : Outport
  wires:
  Demux/4 -> Mux/4  "Vhcl Steering Trq"
  Demux/2 -> Mux/2  "Vhcl Steering AngVel"
  Demux/3 -> Mux/3  "Vhcl Steering AngAcc"
  Demux/1 -> Mux/1  "Vhcl Steering Ang"
  Mux/1 -> Vhcl.Steering/1
  Ground7/1 -> Demux/1

== system generic_uservehicle_truck/TruckMaker/Vehicle/User Vehicle (CM4SL)/CarAndTrailer/CreateBus Vhcl.Wheel.FL ==
  Demux3 : Demux  Outputs=14
  Ground3 : Ground
  Mux : Mux  Inputs=14
  Vhcl.Wheel.FL : Outport
  wires:
  Demux3/1 -> Mux/1  "Vhcl Wheel FL t x"
  Mux/1 -> Vhcl.Wheel.FL/1
  Ground3/1 -> Demux3/1
  Demux3/2 -> Mux/2  "Vhcl Wheel FL t y"
  Demux3/3 -> Mux/3  "Vhcl Wheel FL t z"
  Demux3/4 -> Mux/4  "Vhcl Wheel FL r_zxy x"
  Demux3/5 -> Mux/5  "Vhcl Wheel FL r_zxy y"
  Demux3/6 -> Mux/6  "Vhcl Wheel FL r_zxy z"
  Demux3/7 -> Mux/7  "Vhcl Wheel FL Fx"
  Demux3/8 -> Mux/8  "Vhcl Wheel FL Fy"
  Demux3/9 -> Mux/9  "Vhcl Wheel FL Fz"
  Demux3/10 -> Mux/10  "Vhcl Wheel FL vBelt"
  Demux3/11 -> Mux/11  "Vhcl Wheel FL LongSlip"
  Demux3/12 -> Mux/12  "Vhcl Wheel FL SideSlip"
  Demux3/13 -> Mux/13  "Vhcl Wheel FL Trq_T2W"
  Demux3/14 -> Mux/14  "Vhcl Wheel FL Trq_WhlBearing"

== system generic_uservehicle_truck/TruckMaker/Vehicle/User Vehicle (CM4SL)/CarAndTrailer/CreateBus Vhcl.Wheel.FL2 ==
  Bus Creator3 : BusCreator  Inputs=14
  Demux3 : Demux  Outputs=14
  Ground5 : Ground
  Vhcl.Wheel.FL2 : Outport
  wires:
  Demux3/14 -> Bus Creator3/14  "Vhcl Wheel FL2 Trq_WhlBearing"
  Demux3/13 -> Bus Creator3/13  "Vhcl Wheel FL2 Trq_T2W"
  Demux3/12 -> Bus Creator3/12  "Vhcl Wheel FL2 SideSlip"
  Demux3/11 -> Bus Creator3/11  "Vhcl Wheel FL2 LongSlip"
  Demux3/10 -> Bus Creator3/10  "Vhcl Wheel FL2 vBelt"
  Demux3/9 -> Bus Creator3/9  "Vhcl Wheel FL2 Fz"
  Demux3/8 -> Bus Creator3/8  "Vhcl Wheel FL2 Fy"
  Demux3/7 -> Bus Creator3/7  "Vhcl Wheel FL2 Fx"
  Demux3/6 -> Bus Creator3/6  "Vhcl Wheel FL2 r_zxy z"
  Demux3/5 -> Bus Creator3/5  "Vhcl Wheel FL2 r_zxy y"
  Demux3/4 -> Bus Creator3/4  "Vhcl Wheel FL2 r_zxy x"
  Demux3/3 -> Bus Creator3/3  "Vhcl Wheel FL2 t z"
  Demux3/2 -> Bus Creator3/2  "Vhcl Wheel FL2 t y"
  Demux3/1 -> Bus Creator3/1  "Vhcl Wheel FL2 t x"
  Bus Creator3/1 -> Vhcl.Wheel.FL2/1
  Ground5/1 -> Demux3/1

== system generic_uservehicle_truck/TruckMaker/Vehicle/User Vehicle (CM4SL)/CarAndTrailer/CreateBus Vhcl.Wheel.FR ==
  Demux3 : Demux  Outputs=14
  Ground4 : Ground
  Mux : Mux  Inputs=14
  Vhcl.Wheel.FR : Outport
  wires:
  Demux3/1 -> Mux/1  "Vhcl Wheel FR t x"
  Mux/1 -> Vhcl.Wheel.FR/1
  Ground4/1 -> Demux3/1
  Demux3/2 -> Mux/2  "Vhcl Wheel FR t y"
  Demux3/3 -> Mux/3  "Vhcl Wheel FR t z"
  Demux3/4 -> Mux/4  "Vhcl Wheel FR r_zxy x"
  Demux3/5 -> Mux/5  "Vhcl Wheel FR r_zxy y"
  Demux3/6 -> Mux/6  "Vhcl Wheel FR r_zxy z"
  Demux3/7 -> Mux/7  "Vhcl Wheel FR Fx"
  Demux3/8 -> Mux/8  "Vhcl Wheel FR Fy"
  Demux3/9 -> Mux/9  "Vhcl Wheel FR Fz"
  Demux3/10 -> Mux/10  "Vhcl Wheel FR vBelt"
  Demux3/11 -> Mux/11  "Vhcl Wheel FR LongSlip"
  Demux3/12 -> Mux/12  "Vhcl Wheel FR SideSlip"
  Demux3/13 -> Mux/13  "Vhcl Wheel FR Trq_T2W"
  Demux3/14 -> Mux/14  "Vhcl Wheel FR Trq_WhlBearing"

== system generic_uservehicle_truck/TruckMaker/Vehicle/User Vehicle (CM4SL)/CarAndTrailer/CreateBus Vhcl.Wheel.FR2 ==
  Bus Creator3 : BusCreator  Inputs=14
  Demux3 : Demux  Outputs=14
  Ground6 : Ground
  Vhcl.Wheel.FR2 : Outport
  wires:
  Demux3/14 -> Bus Creator3/14  "Vhcl Wheel FR2 Trq_WhlBearing"
  Demux3/13 -> Bus Creator3/13  "Vhcl Wheel FR2 Trq_T2W"
  Demux3/12 -> Bus Creator3/12  "Vhcl Wheel FR2 SideSlip"
  Demux3/11 -> Bus Creator3/11  "Vhcl Wheel FR2 LongSlip"
  Demux3/10 -> Bus Creator3/10  "Vhcl Wheel FR2 vBelt"
  Demux3/9 -> Bus Creator3/9  "Vhcl Wheel FR2 Fz"
  Demux3/8 -> Bus Creator3/8  "Vhcl Wheel FR2 Fy"
  Demux3/7 -> Bus Creator3/7  "Vhcl Wheel FR2 Fx"
  Demux3/6 -> Bus Creator3/6  "Vhcl Wheel FR2 r_zxy z"
  Demux3/5 -> Bus Creator3/5  "Vhcl Wheel FR2 r_zxy y"
  Demux3/4 -> Bus Creator3/4  "Vhcl Wheel FR2 r_zxy x"
  Demux3/3 -> Bus Creator3/3  "Vhcl Wheel FR2 t z"
  Demux3/2 -> Bus Creator3/2  "Vhcl Wheel FR2 t y"
  Demux3/1 -> Bus Creator3/1  "Vhcl Wheel FR2 t x"
  Bus Creator3/1 -> Vhcl.Wheel.FR2/1
  Ground6/1 -> Demux3/1

== system generic_uservehicle_truck/TruckMaker/Vehicle/User Vehicle (CM4SL)/CarAndTrailer/CreateBus Vhcl.Wheel.RL ==
  Demux3 : Demux  Outputs=14
  Ground5 : Ground
  Mux : Mux  Inputs=14
  Vhcl.Wheel.RL : Outport
  wires:
  Demux3/1 -> Mux/1  "Vhcl Wheel RL t x"
  Mux/1 -> Vhcl.Wheel.RL/1
  Ground5/1 -> Demux3/1
  Demux3/2 -> Mux/2  "Vhcl Wheel RL t y"
  Demux3/3 -> Mux/3  "Vhcl Wheel RL t z"
  Demux3/4 -> Mux/4  "Vhcl Wheel RL r_zxy x"
  Demux3/5 -> Mux/5  "Vhcl Wheel RL r_zxy y"
  Demux3/6 -> Mux/6  "Vhcl Wheel RL r_zxy z"
  Demux3/7 -> Mux/7  "Vhcl Wheel RL Fx"
  Demux3/8 -> Mux/8  "Vhcl Wheel RL Fy"
  Demux3/9 -> Mux/9  "Vhcl Wheel RL Fz"
  Demux3/10 -> Mux/10  "Vhcl Wheel RL vBelt"
  Demux3/11 -> Mux/11  "Vhcl Wheel RL LongSlip"
  Demux3/12 -> Mux/12  "Vhcl Wheel RL SideSlip"
  Demux3/13 -> Mux/13  "Vhcl Wheel RL Trq_T2W"
  Demux3/14 -> Mux/14  "Vhcl Wheel RL Trq_WhlBearing"

== system generic_uservehicle_truck/TruckMaker/Vehicle/User Vehicle (CM4SL)/CarAndTrailer/CreateBus Vhcl.Wheel.RL2 ==
  Bus Creator3 : BusCreator  Inputs=14
  Demux3 : Demux  Outputs=14
  Ground3 : Ground
  Vhcl.Wheel.RL2 : Outport
  wires:
  Bus Creator3/1 -> Vhcl.Wheel.RL2/1
  Demux3/14 -> Bus Creator3/14  "Vhcl Wheel RL2 Trq_WhlBearing"
  Demux3/13 -> Bus Creator3/13  "Vhcl Wheel RL2 Trq_T2W"
  Demux3/12 -> Bus Creator3/12  "Vhcl Wheel RL2 SideSlip"
  Demux3/11 -> Bus Creator3/11  "Vhcl Wheel RL2 LongSlip"
  Demux3/10 -> Bus Creator3/10  "Vhcl Wheel RL2 vBelt"
  Demux3/9 -> Bus Creator3/9  "Vhcl Wheel RL2 Fz"
  Demux3/8 -> Bus Creator3/8  "Vhcl Wheel RL2 Fy"
  Demux3/7 -> Bus Creator3/7  "Vhcl Wheel RL2 Fx"
  Demux3/6 -> Bus Creator3/6  "Vhcl Wheel RL2 r_zxy z"
  Demux3/5 -> Bus Creator3/5  "Vhcl Wheel RL2 r_zxy y"
  Demux3/4 -> Bus Creator3/4  "Vhcl Wheel RL2 r_zxy x"
  Demux3/3 -> Bus Creator3/3  "Vhcl Wheel RL2 t z"
  Demux3/2 -> Bus Creator3/2  "Vhcl Wheel RL2 t y"
  Demux3/1 -> Bus Creator3/1  "Vhcl Wheel RL2 t x"
  Ground3/1 -> Demux3/1

== system generic_uservehicle_truck/TruckMaker/Vehicle/User Vehicle (CM4SL)/CarAndTrailer/CreateBus Vhcl.Wheel.RR ==
  Demux3 : Demux  Outputs=14
  Ground6 : Ground
  Mux : Mux  Inputs=14
  Vhcl.Wheel.RR : Outport
  wires:
  Demux3/1 -> Mux/1  "Vhcl Wheel RR t x"
  Mux/1 -> Vhcl.Wheel.RR/1
  Ground6/1 -> Demux3/1
  Demux3/2 -> Mux/2  "Vhcl Wheel RR t y"
  Demux3/3 -> Mux/3  "Vhcl Wheel RR t z"
  Demux3/4 -> Mux/4  "Vhcl Wheel RR r_zxy x"
  Demux3/5 -> Mux/5  "Vhcl Wheel RR r_zxy y"
  Demux3/6 -> Mux/6  "Vhcl Wheel RR r_zxy z"
  Demux3/7 -> Mux/7  "Vhcl Wheel RR Fx"
  Demux3/8 -> Mux/8  "Vhcl Wheel RR Fy"
  Demux3/9 -> Mux/9  "Vhcl Wheel RR Fz"
  Demux3/10 -> Mux/10  "Vhcl Wheel RR vBelt"
  Demux3/11 -> Mux/11  "Vhcl Wheel RR LongSlip"
  Demux3/12 -> Mux/12  "Vhcl Wheel RR SideSlip"
  Demux3/13 -> Mux/13  "Vhcl Wheel RR Trq_T2W"
  Demux3/14 -> Mux/14  "Vhcl Wheel RR Trq_WhlBearing"

== system generic_uservehicle_truck/TruckMaker/Vehicle/User Vehicle (CM4SL)/CarAndTrailer/CreateBus Vhcl.Wheel.RR2 ==
  Bus Creator3 : BusCreator  Inputs=14
  Demux3 : Demux  Outputs=14
  Ground4 : Ground
  Vhcl.Wheel.RR2 : Outport
  wires:
  Demux3/14 -> Bus Creator3/14  "Vhcl Wheel RR2 Trq_WhlBearing"
  Demux3/13 -> Bus Creator3/13  "Vhcl Wheel RR2 Trq_T2W"
  Demux3/12 -> Bus Creator3/12  "Vhcl Wheel RR2 SideSlip"
  Demux3/11 -> Bus Creator3/11  "Vhcl Wheel RR2 LongSlip"
  Demux3/10 -> Bus Creator3/10  "Vhcl Wheel RR2 vBelt"
  Demux3/9 -> Bus Creator3/9  "Vhcl Wheel RR2 Fz"
  Demux3/8 -> Bus Creator3/8  "Vhcl Wheel RR2 Fy"
  Demux3/7 -> Bus Creator3/7  "Vhcl Wheel RR2 Fx"
  Demux3/6 -> Bus Creator3/6  "Vhcl Wheel RR2 r_zxy z"
  Demux3/5 -> Bus Creator3/5  "Vhcl Wheel RR2 r_zxy y"
  Demux3/4 -> Bus Creator3/4  "Vhcl Wheel RR2 r_zxy x"
  Demux3/3 -> Bus Creator3/3  "Vhcl Wheel RR2 t z"
  Demux3/2 -> Bus Creator3/2  "Vhcl Wheel RR2 t y"
  Demux3/1 -> Bus Creator3/1  "Vhcl Wheel RR2 t x"
  Bus Creator3/1 -> Vhcl.Wheel.RR2/1
  Ground4/1 -> Demux3/1

== system generic_uservehicle_truck/TruckMaker/Vehicle/User Vehicle (ModelMgr)/Brake/CreateBus Vhcl.Wheel.PT ==
  In : Inport
  BusCreator : BusCreator  Inputs=40
  Demux : Demux  Outputs=40
  Out : Outport
  wires:
  Demux/40 -> BusCreator/40  "Vhcl Trq_DriveSrc_trg d7"
  Demux/39 -> BusCreator/39  "Vhcl Trq_DriveSrc_trg d6"
  Demux/38 -> BusCreator/38  "Vhcl Trq_DriveSrc_trg d5"
  Demux/37 -> BusCreator/37  "Vhcl Trq_DriveSrc_trg d4"
  Demux/36 -> BusCreator/36  "Vhcl Trq_DriveSrc_trg d3"
  Demux/35 -> BusCreator/35  "Vhcl Trq_DriveSrc_trg d2"
  Demux/34 -> BusCreator/34  "Vhcl Trq_DriveSrc_trg d1"
  Demux/33 -> BusCreator/33  "Vhcl Trq_DriveSrc_trg d0"
  Demux/32 -> BusCreator/32  "Vhcl Wheel FR2 WhlBearing"
  Demux/31 -> BusCreator/31  "Vhcl Wheel FR2 Trq_T2W"
  Demux/30 -> BusCreator/30  "Vhcl Wheel FR2 Trq_BrakeReg_trg"
  Demux/29 -> BusCreator/29  "Vhcl Wheel FR2 Trq_Brake"
  Demux/28 -> BusCreator/28  "Vhcl Wheel FL2 WhlBearing"
  Demux/27 -> BusCreator/27  "Vhcl Wheel FL2 Trq_T2W"
  Demux/26 -> BusCreator/26  "Vhcl Wheel FL2 Trq_BrakeReg_trg"
  Demux/25 -> BusCreator/25  "Vhcl Wheel FL2 Trq_Brake"
  Demux/24 -> BusCreator/24  "Vhcl Wheel RR2 WhlBearing"
  Demux/23 -> BusCreator/23  "Vhcl Wheel RR2 Trq_T2W"
  Demux/22 -> BusCreator/22  "Vhcl Wheel RR2 Trq_BrakeReg_trg"
  Demux/21 -> BusCreator/21  "Vhcl Wheel RR2 Trq_Brake"
  Demux/20 -> BusCreator/20  "Vhcl Wheel RL2 WhlBearing"
  Demux/19 -> BusCreator/19  "Vhcl Wheel RL2 Trq_T2W"
  Demux/18 -> BusCreator/18  "Vhcl Wheel RL2 Trq_BrakeReg_trg"
  Demux/17 -> BusCreator/17  "Vhcl Wheel RL2 Trq_Brake"
  Demux/16 -> BusCreator/16  "Vhcl Wheel RR WhlBearing"
  Demux/15 -> BusCreator/15  "Vhcl Wheel RR Trq_T2W"
  Demux/14 -> BusCreator/14  "Vhcl Wheel RR Trq_BrakeReg_trg"
  Demux/13 -> BusCreator/13  "Vhcl Wheel RR Trq_Brake"
  Demux/12 -> BusCreator/12  "Vhcl Wheel RL WhlBearing"
  Demux/11 -> BusCreator/11  "Vhcl Wheel RL Trq_T2W"
  Demux/10 -> BusCreator/10  "Vhcl Wheel RL Trq_BrakeReg_trg"
  Demux/9 -> BusCreator/9  "Vhcl Wheel RL Trq_Brake"
  Demux/8 -> BusCreator/8  "Vhcl Wheel FR WhlBearing"
  Demux/7 -> BusCreator/7  "Vhcl Wheel FR Trq_T2W"
  Demux/6 -> BusCreator/6  "Vhcl Wheel FR Trq_BrakeReg_trg"
  Demux/5 -> BusCreator/5  "Vhcl Wheel FR Trq_Brake"
  Demux/4 -> BusCreator/4  "Vhcl Wheel FL WhlBearing"
  Demux/3 -> BusCreator/3  "Vhcl Wheel FL Trq_T2W"
  Demux/2 -> BusCreator/2  "Vhcl Wheel FL Trq_BrakeReg_trg"
  Demux/1 -> BusCreator/1  "Vhcl Wheel FL Trq_Brake"
  BusCreator/1 -> Out/1
  In/1 -> Demux/1

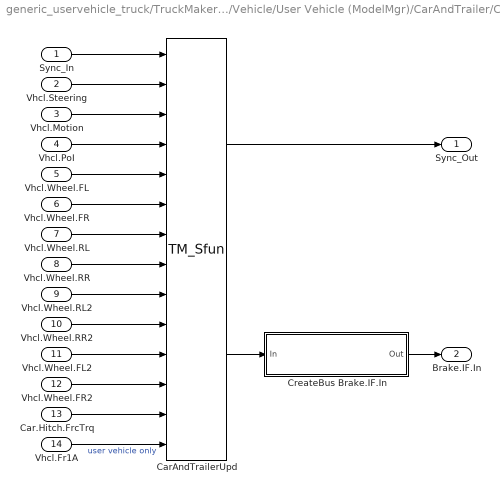
== system generic_uservehicle_truck/TruckMaker/Vehicle/User Vehicle (ModelMgr)/CarAndTrailer/CarAndTrailerUpd ==
  Sync_In : Inport
  Vhcl.Steering : Inport  Port=2
  Vhcl.Motion : Inport  Port=3
  Vhcl.PoI : Inport  Port=4
  Vhcl.Wheel.FL : Inport  Port=5
  Vhcl.Wheel.FR : Inport  Port=6
  Vhcl.Wheel.RL : Inport  Port=7
  Vhcl.Wheel.RR : Inport  Port=8
  Vhcl.Wheel.RL2 : Inport  Port=9
  Vhcl.Wheel.RR2 : Inport  Port=10
  Vhcl.Wheel.FL2 : Inport  Port=11
  Vhcl.Wheel.FR2 : Inport  Port=12
  Car.Hitch.FrcTrq : Inport  Port=13
  Vhcl.Fr1A : Inport  Port=14
  CarAndTrailerUpd : S-Function  FunctionName=TM_Sfun  Parameters='CarAndTrUpd'  SFunctionDeploymentMode=off  EnableBusSupport=off
  CreateBus Brake.IF.In : Subsystem
  Sync_Out : Outport
  Brake.IF.In : Outport  Port=2
  wires:
  Vhcl.Fr1A/1 -> CarAndTrailerUpd/14  "user vehicle only"
  Vhcl.Wheel.RL2/1 -> CarAndTrailerUpd/9
  Vhcl.Wheel.RR2/1 -> CarAndTrailerUpd/10
  Vhcl.Wheel.FL2/1 -> CarAndTrailerUpd/11
  Vhcl.Wheel.FR2/1 -> CarAndTrailerUpd/12
  Car.Hitch.FrcTrq/1 -> CarAndTrailerUpd/13
  Vhcl.Wheel.RR/1 -> CarAndTrailerUpd/8
  Vhcl.Wheel.RL/1 -> CarAndTrailerUpd/7
  Vhcl.Wheel.FR/1 -> CarAndTrailerUpd/6
  Vhcl.Wheel.FL/1 -> CarAndTrailerUpd/5
  Vhcl.Steering/1 -> CarAndTrailerUpd/2
  Vhcl.Motion/1 -> CarAndTrailerUpd/3
  Vhcl.PoI/1 -> CarAndTrailerUpd/4
  CarAndTrailerUpd/2 -> CreateBus Brake.IF.In/1(In)
  CreateBus Brake.IF.In/1(Out) -> Brake.IF.In/1
  CarAndTrailerUpd/1 -> Sync_Out/1
  Sync_In/1 -> CarAndTrailerUpd/1

== system generic_uservehicle_truck/TruckMaker/Vehicle/IPG Vehicle/CarAndTrailer/CarAndTrailerUpd/CreateBus Brake.IF.In ==
  In : Inport
  BusCreator : BusCreator  Inputs=17
  Demux : Demux  Outputs=17
  Out : Outport
  wires:
  Demux/17 -> BusCreator/17  "Brake IF Trq_Reg FR2"
  Demux/16 -> BusCreator/16  "Brake IF Trq_Reg FL2"
  Demux/15 -> BusCreator/15  "Brake IF Trq_Reg RR2"
  Demux/14 -> BusCreator/14  "Brake IF Trq_Reg RL2"
  Demux/13 -> BusCreator/13  "Brake IF Trq_Reg RR"
  Demux/12 -> BusCreator/12  "Brake IF Trq_Reg RL"
  Demux/11 -> BusCreator/11  "Brake IF Trq_Reg FR"
  Demux/10 -> BusCreator/10  "Brake IF Trq_Reg FL"
  Demux/9 -> BusCreator/9  "Brake IF Trq_Reg_max FR2"
  Demux/8 -> BusCreator/8  "Brake IF Trq_Reg_max FL2"
  Demux/7 -> BusCreator/7  "Brake IF Trq_Reg_max RR2"
  Demux/6 -> BusCreator/6  "Brake IF Trq_Reg_max RL2"
  Demux/5 -> BusCreator/5  "Brake IF Trq_Reg_max RR"
  Demux/4 -> BusCreator/4  "Brake IF Trq_Reg_max RL"
  Demux/3 -> BusCreator/3  "Brake IF Trq_Reg_max FR"
  Demux/2 -> BusCreator/2  "Brake IF Trq_Reg_max FL"
  Demux/1 -> BusCreator/1  "Brake IF T_env"
  BusCreator/1 -> Out/1
  In/1 -> Demux/1

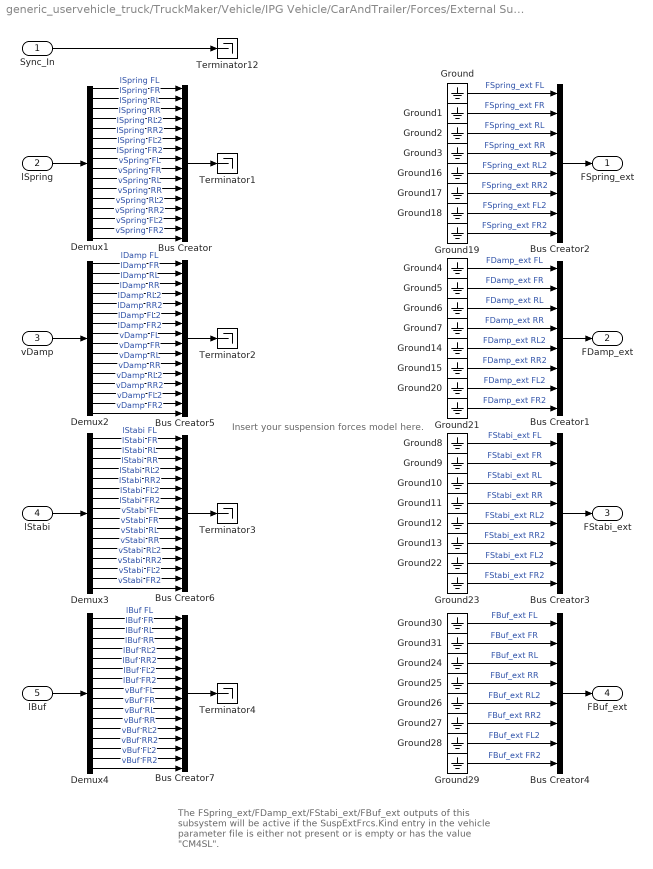
== system generic_uservehicle_truck/TruckMaker/Vehicle/IPG Vehicle/CarAndTrailer/Forces/External Suspension Forces ==
  note: The FSpring_ext/FDamp_ext/FStabi_ext/FBuf_ext outputs of this subsystem will be
      | active if the SuspExtFrcs.Kind entry in the vehicle parameter file
      | is either not present or is empty or has the value "CM4SL".
  note: Insert your suspension forces model here.
  Sync_In : Inport
  lSpring : Inport  Port=2
  vDamp : Inport  Port=3
  lStabi : Inport  Port=4
  lBuf : Inport  Port=5
  Bus Creator{,5..7} (4 alike) : BusCreator  Inputs=16
  Bus Creator{1..4} (4 alike) : BusCreator  Inputs=8
  Demux{1..4} (4 alike) : Demux  Outputs=16
  Ground{,1..31} (32 alike) : Ground
  Terminator{1..4,12} (5 alike) : Terminator
  FSpring_ext : Outport
  FDamp_ext : Outport  Port=2
  FStabi_ext : Outport  Port=3
  FBuf_ext : Outport  Port=4
  wires:
  Demux3/10 -> Bus Creator6/10  "vStabi FR"
  Demux4/16 -> Bus Creator7/16  "vBuf FR2"
  Demux4/15 -> Bus Creator7/15  "vBuf FL2"
  Demux4/14 -> Bus Creator7/14  "vBuf RR2"
  Demux4/13 -> Bus Creator7/13  "vBuf RL2"
  Demux4/12 -> Bus Creator7/12  "vBuf RR"
  Demux4/11 -> Bus Creator7/11  "vBuf RL"
  Demux4/10 -> Bus Creator7/10  "vBuf FR"
  Demux4/9 -> Bus Creator7/9  "vBuf FL"
  Demux3/16 -> Bus Creator6/16  "vStabi FR2"
  Demux3/15 -> Bus Creator6/15  "vStabi FL2"
  Demux3/14 -> Bus Creator6/14  "vStabi RR2"
  Demux3/13 -> Bus Creator6/13  "vStabi RL2"
  Demux3/12 -> Bus Creator6/12  "vStabi RR"
  Demux3/11 -> Bus Creator6/11  "vStabi RL"
  Demux3/9 -> Bus Creator6/9  "vStabi FL"
  Bus Creator6/1 -> Terminator3/1
  Bus Creator7/1 -> Terminator4/1
  Bus Creator5/1 -> Terminator2/1
  Bus Creator/1 -> Terminator1/1
  Demux2/16 -> Bus Creator5/16  "vDamp FR2"
  Demux2/15 -> Bus Creator5/15  "vDamp FL2"
  Demux2/14 -> Bus Creator5/14  "vDamp RR2"
  Demux2/13 -> Bus Creator5/13  "vDamp RL2"
  Demux2/12 -> Bus Creator5/12  "vDamp RR"
  Demux2/11 -> Bus Creator5/11  "vDamp RL"
  Demux2/10 -> Bus Creator5/10  "vDamp FR"
  Demux2/9 -> Bus Creator5/9  "vDamp FL"
  Demux1/16 -> Bus Creator/16  "vSpring FR2"
  Demux1/15 -> Bus Creator/15  "vSpring FL2"
  Demux1/14 -> Bus Creator/14  "vSpring RR2"
  Demux1/13 -> Bus Creator/13  "vSpring RL2"
  Demux1/12 -> Bus Creator/12  "vSpring RR"
  Demux1/11 -> Bus Creator/11  "vSpring RL"
  Demux1/10 -> Bus Creator/10  "vSpring FR"
  Demux1/9 -> Bus Creator/9  "vSpring FL"
  Demux3/7 -> Bus Creator6/7  "lStabi FL2"
  Demux3/8 -> Bus Creator6/8  "lStabi FR2"
  Ground22/1 -> Bus Creator3/7  "FStabi_ext FL2"
  Ground23/1 -> Bus Creator3/8  "FStabi_ext FR2"
  Demux2/7 -> Bus Creator5/7  "lDamp FL2"
  Demux2/8 -> Bus Creator5/8  "lDamp FR2"
  Ground20/1 -> Bus Creator1/7  "FDamp_ext FL2"
  Ground21/1 -> Bus Creator1/8  "FDamp_ext FR2"
  Ground18/1 -> Bus Creator2/7  "FSpring_ext FL2"
  Ground19/1 -> Bus Creator2/8  "FSpring_ext FR2"
  Demux1/7 -> Bus Creator/7  "lSpring FL2"
  Demux1/8 -> Bus Creator/8  "lSpring FR2"
  Sync_In/1 -> Terminator12/1
  lSpring/1 -> Demux1/1
  vDamp/1 -> Demux2/1
  lStabi/1 -> Demux3/1
  Demux3/1 -> Bus Creator6/1  "lStabi FL"
  Demux3/2 -> Bus Creator6/2  "lStabi FR"
  Demux3/3 -> Bus Creator6/3  "lStabi RL"
  Demux3/4 -> Bus Creator6/4  "lStabi RR"
  Demux1/1 -> Bus Creator/1  "lSpring FL"
  Demux1/2 -> Bus Creator/2  "lSpring FR"
  Demux1/3 -> Bus Creator/3  "lSpring RL"
  Demux1/4 -> Bus Creator/4  "lSpring RR"
  Demux2/1 -> Bus Creator5/1  "lDamp FL"
  Demux2/2 -> Bus Creator5/2  "lDamp FR"
  Demux2/3 -> Bus Creator5/3  "lDamp RL"
  Demux2/4 -> Bus Creator5/4  "lDamp RR"
  Bus Creator2/1 -> FSpring_ext/1
  Ground/1 -> Bus Creator2/1  "FSpring_ext FL"
  Ground1/1 -> Bus Creator2/2  "FSpring_ext FR"
  Ground2/1 -> Bus Creator2/3  "FSpring_ext RL"
  Ground3/1 -> Bus Creator2/4  "FSpring_ext RR"
  Ground4/1 -> Bus Creator1/1  "FDamp_ext FL"
  Ground5/1 -> Bus Creator1/2  "FDamp_ext FR"
  Ground6/1 -> Bus Creator1/3  "FDamp_ext RL"
  Ground7/1 -> Bus Creator1/4  "FDamp_ext RR"
  Bus Creator1/1 -> FDamp_ext/1
  Ground8/1 -> Bus Creator3/1  "FStabi_ext FL"
  Ground9/1 -> Bus Creator3/2  "FStabi_ext FR"
  Ground10/1 -> Bus Creator3/3  "FStabi_ext RL"
  Ground11/1 -> Bus Creator3/4  "FStabi_ext RR"
  Bus Creator3/1 -> FStabi_ext/1
  Demux3/5 -> Bus Creator6/5  "lStabi RL2"
  Demux3/6 -> Bus Creator6/6  "lStabi RR2"
  Ground12/1 -> Bus Creator3/5  "FStabi_ext RL2"
  Ground13/1 -> Bus Creator3/6  "FStabi_ext RR2"
  Demux2/5 -> Bus Creator5/5  "lDamp RL2"
  Demux2/6 -> Bus Creator5/6  "lDamp RR2"
  Ground14/1 -> Bus Creator1/5  "FDamp_ext RL2"
  Ground15/1 -> Bus Creator1/6  "FDamp_ext RR2"
  Demux1/5 -> Bus Creator/5  "lSpring RL2"
  Demux1/6 -> Bus Creator/6  "lSpring RR2"
  Ground16/1 -> Bus Creator2/5  "FSpring_ext RL2"
  Ground17/1 -> Bus Creator2/6  "FSpring_ext RR2"
  Demux4/7 -> Bus Creator7/7  "lBuf FL2"
  Demux4/8 -> Bus Creator7/8  "lBuf FR2"
  Ground28/1 -> Bus Creator4/7  "FBuf_ext FL2"
  Ground29/1 -> Bus Creator4/8  "FBuf_ext FR2"
  lBuf/1 -> Demux4/1
  Demux4/1 -> Bus Creator7/1  "lBuf FL"
  Demux4/2 -> Bus Creator7/2  "lBuf FR"
  Demux4/3 -> Bus Creator7/3  "lBuf RL"
  Demux4/4 -> Bus Creator7/4  "lBuf RR"
  Ground30/1 -> Bus Creator4/1  "FBuf_ext FL"
  Ground31/1 -> Bus Creator4/2  "FBuf_ext FR"
  Ground24/1 -> Bus Creator4/3  "FBuf_ext RL"
  Ground25/1 -> Bus Creator4/4  "FBuf_ext RR"
  Bus Creator4/1 -> FBuf_ext/1
  Demux4/5 -> Bus Creator7/5  "lBuf RL2"
  Demux4/6 -> Bus Creator7/6  "lBuf RR2"
  Ground26/1 -> Bus Creator4/5  "FBuf_ext RL2"
  Ground27/1 -> Bus Creator4/6  "FBuf_ext RR2"
